simulink model "KalmanFilter"  (R2021a)
settings: Solver=VariableStepAuto  StartTime=0.0  StopTime=10.0  RelTol=1e-3
undefined symbols (not defined in the file): A, B, C1
settings Model: Creator=vedan  LastModifiedBy=vedan

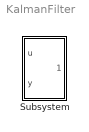
== system KalmanFilter ==
  Subsystem : Subsystem

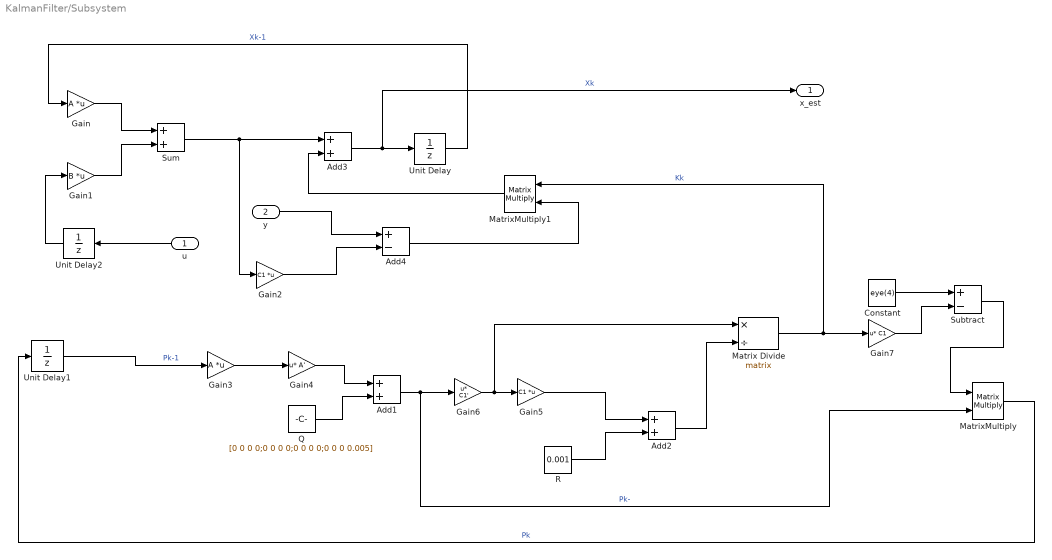
== system KalmanFilter/Subsystem ==
  u : Inport
  y : Inport  Port=2
  Add1 : Sum
  Add2 : Sum
  Add3 : Sum
  Add4 : Sum  Inputs=+-
  Constant : Constant  Value=eye(4)
  Gain : Gain  Gain=A  Multiplication=Matrix(K*u)
  Gain1 : Gain  Gain=B  Multiplication=Matrix(K*u)
  Gain2 : Gain  Gain=C1  Multiplication=Matrix(K*u)
  Gain3 : Gain  Gain=A  Multiplication=Matrix(K*u)
  Gain4 : Gain  Gain=A'  Multiplication=Matrix(u*K)
  Gain5 : Gain  Gain=C1  Multiplication=Matrix(K*u)
  Gain6 : Gain  Gain=C1'  Multiplication=Matrix(u*K)
  Gain7 : Gain  Gain=C1  Multiplication=Matrix(u*K)
  Matrix Divide : Product  Inputs=*/  Multiplication=Matrix(*)
  MatrixMultiply : Product  Multiplication=Matrix(*)
  MatrixMultiply1 : Product  Multiplication=Matrix(*)
  Q : Constant  Value=[0 0 0 0;0 0 0 0;0 0 0 0;0 0 0 0.005]
  R : Constant  Value=0.001
  Subtract : Sum  Inputs=+-
  Sum : Sum
  Unit Delay : UnitDelay  InitialCondition=[0;1;0;0]  SampleTime=0.01  HasFrameUpgradeWarning=on
  Unit Delay1 : UnitDelay  SampleTime=0.01  HasFrameUpgradeWarning=on
  Unit Delay2 : UnitDelay  SampleTime=-1  HasFrameUpgradeWarning=on
  x_est : Outport
  wires:
  Add2/1 -> Matrix Divide/2
  Add4/1 -> MatrixMultiply1/2
  Sum/1 -> Gain2/1, Add3/1
  Gain4/1 -> Add1/1
  Add3/1 -> x_est/1, Unit Delay/1  "Xk"
  Gain6/1 -> Matrix Divide/1, Gain5/1
  Add1/1 -> MatrixMultiply/2, Gain6/1  "Pk-"
  Q/1 -> Add1/2
  Gain/1 -> Sum/1
  Gain7/1 -> Subtract/2
  Matrix Divide/1 -> MatrixMultiply1/1, Gain7/1  "Kk"
  Unit Delay1/1 -> Gain3/1  "Pk-1"
  Subtract/1 -> MatrixMultiply/1
  Unit Delay2/1 -> Gain1/1
  Gain3/1 -> Gain4/1
  Gain1/1 -> Sum/2
  MatrixMultiply1/1 -> Add3/2
  y/1 -> Add4/1
  MatrixMultiply/1 -> Unit Delay1/1  "Pk"
  R/1 -> Add2/2
  u/1 -> Unit Delay2/1
  Unit Delay/1 -> Gain/1  "Xk-1"
  Gain5/1 -> Add2/1
  Gain2/1 -> Add4/2
  Constant/1 -> Subtract/1
